simulink model "example_HeatingCircuitWithMixerThermostatic"  (R2018b)
settings: Solver=ode45  StartTime=0.0  StopTime=400  RelTol=1e-3
undefined symbols (not defined in the file): path_carnot
libraries: carnot x11, simulink x1
settings Model: Creator=drhf  LastModifiedBy=P41573
settings SFSimCC: SimUseLocalCustomCode=off
settings RTWCC: RTWUseLocalCustomCode=off
settings CodeAppCC: StateflowObjectComments=on

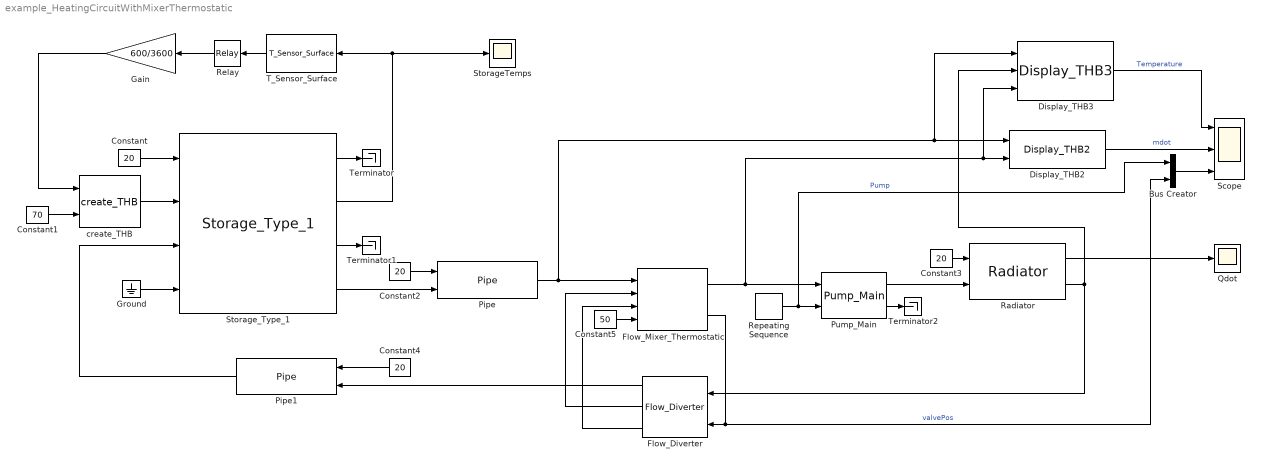
== system example_HeatingCircuitWithMixerThermostatic ==
  Bus Creator : BusCreator  Inputs=2
  Constant{,2..4} (4 alike) : Constant  Value=20
  Constant1 : Constant  Value=70
  Constant5 : Constant  Value=50
  Display_THB2 : carnot/Outputs/Display_THB2  t=off  m=on  p=off  id=off  mix=off  d=off
      settings: SourceProductName=Carnot
  Display_THB3 : carnot/Outputs/Display_THB3  t=on  m=off  p=off  id=off  mix=off  d=off
      settings: SourceProductName=Carnot
  Flow_Diverter : carnot/Hydraulics/Flow_Diverter
      settings: SourceProductName=Carnot
  Flow_Mixer_Thermostatic : carnot/Hydraulics/Flow_Mixer_Thermostatic  t=10
      settings: SourceProductName=Carnot
  Gain : Gain  Gain=600/3600
  Ground : Ground
  Pipe : carnot/Hydraulics/Pipe  dia=0.025  len=10  hgt=0  uloss=100/20/10  cond=0  cwall=1000  t0=20  lin=10  qua=10  nodes=10
      settings: SourceProductName=Carnot
  Pipe1 : carnot/Hydraulics/Pipe  dia=0.025  len=10  hgt=0  uloss=100/20/10  cond=0  cwall=1000  t0=20  lin=10  qua=10  nodes=10
      settings: SourceProductName=Carnot
  Pump_Main : carnot/Hydraulics/Pump_Main  Tini=20  p0=3e5  IDpreset=pressure drop  fluid=Water  mix=0  mix2=0  mix3=0  t1=5  PathName=fullfile(path_carnot('libsl'), 'Hydraulics', 'Pump_Main', 'parameter_set')  FileName='Pump6m.mat'  userPath=off  userParam=off  a0=60000  a1=-43200  a2=0  dia=0.025  UA=1  mcp=4182  e0=50  e1=28.8  e2=-10.368
      settings: SourceProductName=Carnot
  Qdot : Scope
  Radiator : carnot/Source/Heat_Exchanger/Radiator  pnom=5000  dtnom=49.83  expo=1.3  mcap=5*4182  tini=20  lin=10  qua=10
      settings: SourceProductName=Carnot
  Relay : Relay  OnSwitchValue=70  OffSwitchValue=60  OnOutputValue=0  OffOutputValue=1
  Repeating Sequence : simulink/Sources/Repeating Sequence  rep_seq_t=[0 20 60 200]  rep_seq_y=[0 0 1 1]
  Scope : Scope  NumInputPorts=3
  StorageTemps : Scope
  Storage_Type_1 : carnot/Storage/Thermal/Storage_Type_1  t0=70  hgt=1.7684  stgtype=1  tini=[70 70 70 70 70 70 70 70 70 70]  mpts=[1 2 3 4 5 6 7 8 9 10]  PathName=fullfile(path_carnot('libsl'),'Storage','Thermal','Storage_Type_1','parameter_set')  FileName='StorageType1_500_L.mat'  userPath=off  userParam=off  uwall=1  ubot=1  utop=1  axcond=1  volume=0.5  dia=0.6  standing=standing cylinder  nodes=10  mpoints=10  Tsensor=0.5  pipe1inlet=1  pipe1outlet=0  pipe1dia=0.03  pipe2inlet=0  pipe2outlet=1  pipe2dia=0.03  heater1start=0.6  heater1end=0.65
      settings: SourceProductName=Carnot
  T_Sensor_Surface : carnot/Control/T_Sensor_Surface  pos=0.5  tdel=1  t0=70
      settings: SourceProductName=Carnot
  Terminator : Terminator
  Terminator1 : Terminator
  Terminator2 : Terminator
  create_THB : carnot/Source/Simple/create_THB  p=1e5  fluid=Water  mix=0  mix2=0  mix3=0  dia=0  hgt=0  mID=No Pressure Drop
      settings: SourceProductName=Carnot
  wires:
  Constant/1 -> Storage_Type_1/1
  Storage_Type_1/1 -> Terminator/1
  Storage_Type_1/3 -> Terminator1/1
  Storage_Type_1/2 -> StorageTemps/1, T_Sensor_Surface/1
  create_THB/1 -> Storage_Type_1/2
  Constant1/1 -> create_THB/2
  T_Sensor_Surface/1 -> Relay/1
  Relay/1 -> Gain/1
  Gain/1 -> create_THB/1
  Constant2/1 -> Pipe/1
  Pump_Main/2 -> Terminator2/1
  Pipe/1 -> Flow_Mixer_Thermostatic/1, Display_THB3/1, Display_THB2/1
  Repeating Sequence/1 -> Bus Creator/1, Pump_Main/2  "Pump"
  Pump_Main/1 -> Radiator/2
  Radiator/1 -> Qdot/1
  Radiator/2 -> Flow_Diverter/1, Display_THB3/2
  Constant3/1 -> Radiator/1
  Display_THB2/1 -> Scope/2  "mdot"
  Storage_Type_1/4 -> Pipe/2
  Constant4/1 -> Pipe1/1
  Pipe1/1 -> Storage_Type_1/3
  Flow_Diverter/1 -> Pipe1/2
  Flow_Diverter/2 -> Flow_Mixer_Thermostatic/2
  Flow_Diverter/3 -> Flow_Mixer_Thermostatic/3
  Flow_Mixer_Thermostatic/2 -> Flow_Diverter/2, Bus Creator/2  "valvePos"
  Flow_Mixer_Thermostatic/1 -> Display_THB2/2, Display_THB3/3, Pump_Main/1
  Bus Creator/1 -> Scope/3
  Constant5/1 -> Flow_Mixer_Thermostatic/4
  Display_THB3/1 -> Scope/1  "Temperature"
  Ground/1 -> Storage_Type_1/4
